simulink model "CARTESIAN_SPACE"  (R2021a)
settings: Solver=FixedStepAuto  StartTime=0.0  StopTime=10  FixedStep=0.01  RelTol=1e-3
model workspace: external: MATLAB File D:\OneDrive\STUDY\RIC LAB\PROJECT 6DOF\CODE\CODE 6DOF\10_SIMSCAPE\03\ROBOT_DataFile.m (data not in the file)
values from neighbouring files (symbols this model uses):
  circle = zeros(10/step+1,7)    [CIRCLE_01.m]
undefined symbols (not defined in the file or in its folder): smiData, X, Y, Z
libraries: sm_lib x36, nesl_utility x13
(part 1 of 3)
settings Model: Creator=TMP  LastModifiedBy=TMP
settings DataIOCC: SaveTime=off  ReturnWorkspaceOutputs=off
settings ExplorerConfigSet: InternalSimMechanicsExplorerSettings="<ExplorerConfiguration><canonicalview>default</canonicalview><AnimationSetting><BasePlaybackSpeed>1.0</BasePlaybackSpeed><PlaybackSpeedFactor>1.0</PlaybackSpeedFactor></AnimationSetting><TilePanel><TileInfo><Tiles Columns=\"1\" Count=\"1\" Rows=\"1\"><Column Weight=\"1\"/><Row Weight=\"1\"/><Tile Height=\"1\" Width=\"1\" X=\"0\" Y=\"0\"/></Tiles></TileInfo><SceneInfo><SceneViewer><BGColor><R>1</R><G>1</G><B>1</B></BGColor><Camera><DoPerspective>off</DoPerspective><Position><X>0.681216124656701338</X><Y>-0.557879879165802839</Y><Z>0.953804667446790155</Z></Position><Center><X>0.103865855467075482</X><Y>0.0194703900238230587</Y><Z>0.37645439825716448</Z></Center><Up><X>-0.408248290463863073</X><Y>0.408248290463863073</Y><Z>0.816496580927726145</Z></Up><ViewLimDist>1</ViewLimDist><YLim>0.364778303503990209</YLim><XLim>0.455454728380692286</XLim></Camera></SceneViewer></SceneInfo></TilePanel><MechEditorPanel><Cameras/><GfxPanelCameraMap/><VideoCreator><PlaybackSpeedRatio>1.0</PlaybackSpeedRatio><FrameRate>60</FrameRate><VideoFormat>Uncompressed AVI</VideoFormat><FrameSize>[800 600]</FrameSize></VideoCreator></MechEditorPanel></ExplorerConfiguration>"

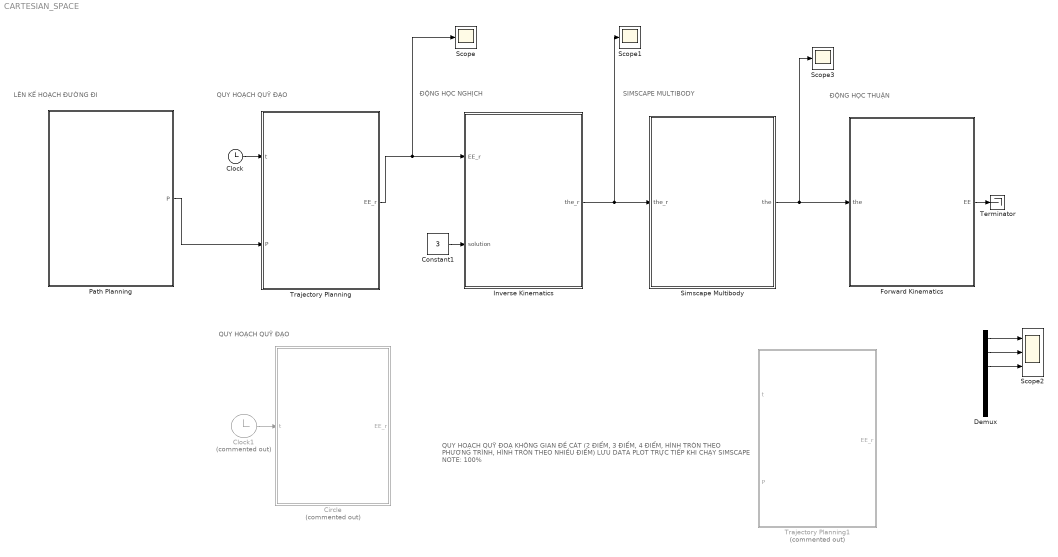
== system CARTESIAN_SPACE ==
  note: QUY HOẠCH QUỸ ĐOẠ KHÔNG GIAN ĐỀ CÁT (2 ĐIỂM, 3 ĐIỂM, 4 ĐIỂM, HÌNH TRÒN THEO PHƯƠNG TRÌNH, HÌNH TRÒN THEO NHIỀU ĐIỂM)
      | LƯU DATA PLOT TRỰC TIẾP KHI CHẠY SIMSCAPE
      | NOTE: 100%
  note: ĐỘNG HỌC NGHỊCH
  note: QUY HOẠCH QUỸ ĐẠO
  note: LÊN KẾ HOẠCH ĐƯỜNG ĐI
  note: QUY HOẠCH QUỸ ĐẠO
  note: SIMSCAPE MULTIBODY
  note: ĐỘNG HỌC THUẬN
  Circle : MATLAB Function  Commented=on  TreatAsAtomicUnit=on
  Clock : Clock
  Clock1 : Clock  Commented=on
  Constant1 : Constant  Value=3
  Demux : Demux  Outputs=6
  Forward Kinematics : MATLAB Function  TreatAsAtomicUnit=on
  Inverse Kinematics : MATLAB Function  TreatAsAtomicUnit=on
  Path Planning : Subsystem
  Scope : Scope
  Scope1 : Scope
  Scope2 : Scope  NumInputPorts=3
  Scope3 : Scope
  Simscape Multibody : Subsystem
  Terminator : Terminator
  Trajectory Planning : MATLAB Function  TreatAsAtomicUnit=on
  Trajectory Planning1 : MATLAB Function  Commented=on  TreatAsAtomicUnit=on
  wires:
  Constant1/1 -> Inverse Kinematics/2(solution)
  Clock1/1 -> Circle/1(t)
  Demux/1 -> Scope2/1
  Demux/2 -> Scope2/2
  Demux/3 -> Scope2/3
  Clock/1 -> Trajectory Planning/1(t)
  Path Planning/1(P) -> Trajectory Planning/2(P)
  Trajectory Planning/1(EE_r) -> Scope/1, Inverse Kinematics/1(EE_r)
  Inverse Kinematics/1(the_r) -> Scope1/1, Simscape Multibody/1(the_r)
  Simscape Multibody/1(the) -> Scope3/1, Forward Kinematics/1(the)
  Forward Kinematics/1(EE) -> Terminator/1

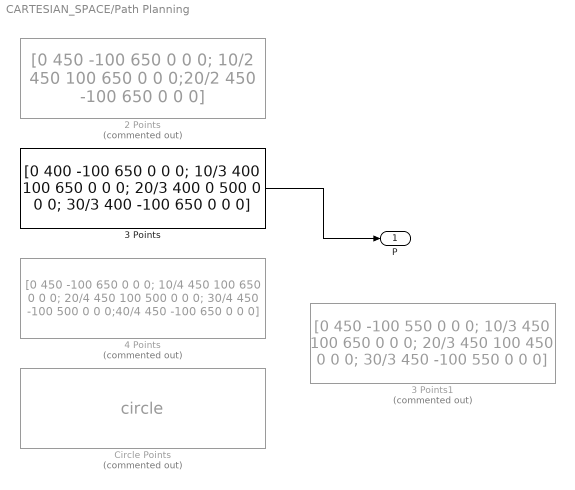
== system CARTESIAN_SPACE/Path Planning ==
  2 Points : Constant  Commented=on  Value=[0 450 -100 650 0 0 0; 10/2 450 100 650 0 0 0;20/2 450 -100 650 0 0 0]
  3 Points : Constant  Value=[0 400 -100 650 0 0 0; 10/3 400 100 650 0 0 0; 20/3 400 0 500 0 0 0; 30/3 400 -100 650 0 0 0]
  3 Points1 : Constant  Commented=on  Value=[0 450 -100 550 0 0 0; 10/3 450 100 650 0 0 0; 20/3 450 100 450 0 0 0; 30/3 450 -100 550 0 0 0]
  4 Points : Constant  Commented=on  Value=[0 450 -100 650 0 0 0; 10/4 450 100 650 0 0 0; 20/4 450 100 500 0 0 0; 30/4 450 -100 500 0 0 0;40/4 450 -100 650 0 0 0]
  Circle Points : Constant  Commented=on  Value=circle
  P : Outport
  wires:
  3 Points/1 -> P/1
